simulink model "MotorSpeedAnalysisLAST"  (R2016a)
settings: Solver=ode4  SolverMode=SingleTasking  StartTime=0.0  StopTime=10  FixedStep=Ts  RelTol=1e-3
undefined symbols (not defined in the file): Ts
libraries: arduino_io_lib x4, powerlib_meascontrol x1
settings Model: ExtModeTrigDuration=2  Creator=gcampa  LastModifiedBy=User
settings DataIOCC: LimitDataPoints=on  SaveFormat=Array  SignalLoggingSaveFormat=ModelDataLogs
settings OptimizationCC: OptimizeModelRefInitCode=on  LifeSpan=1  MaxStackSize=64
settings DebuggingCC: UnderspecifiedInitializationDetection=Classic  MergeDetectMultiDrivingBlocksExec=none  MultiTaskDSMMsg=warning  MultiTaskCondExecSysMsg=none
settings HardwareCC: ProdBitPerInt=16  ProdBitPerPointer=16  ProdLargestAtomicFloat=None  ProdWordSize=8  ProdHWDeviceType=Atmel->AVR
settings ModelReferenceCC: PropagateSignalLabelsOutOfModel=off
settings RTWCC: SystemTargetFile=ert.tlc  HardwareBoard=Arduino Uno  TemplateMakefile=ert_default_tmf  GenerateReport=on  RTWVerbose=off  Toolchain=Arduino AVR v1.6.1  BuildConfiguration=Faster Runs  IncludeHyperlinkInReport=on  LaunchReport=on  GenerateTraceInfo=on  GenerateTraceReport=on  GenerateTraceReportSl=on  GenerateTraceReportSf=on  GenerateTraceReportEml=on
settings CodeAppCC: ForceParamTrailComments=on  IgnoreCustomStorageClasses=off  OperatorAnnotations=on  SimulinkDataObjDesc=on  SFDataObjDesc=on  MATLABFcnDesc=on  InsertBlockDesc=on  MATLABSourceComments=on
settings ERTTargetCC: SupportContinuousTime=on  SupportVariableSizeSignals=on
settings ConfigComp: CovModelRefEnable=Off

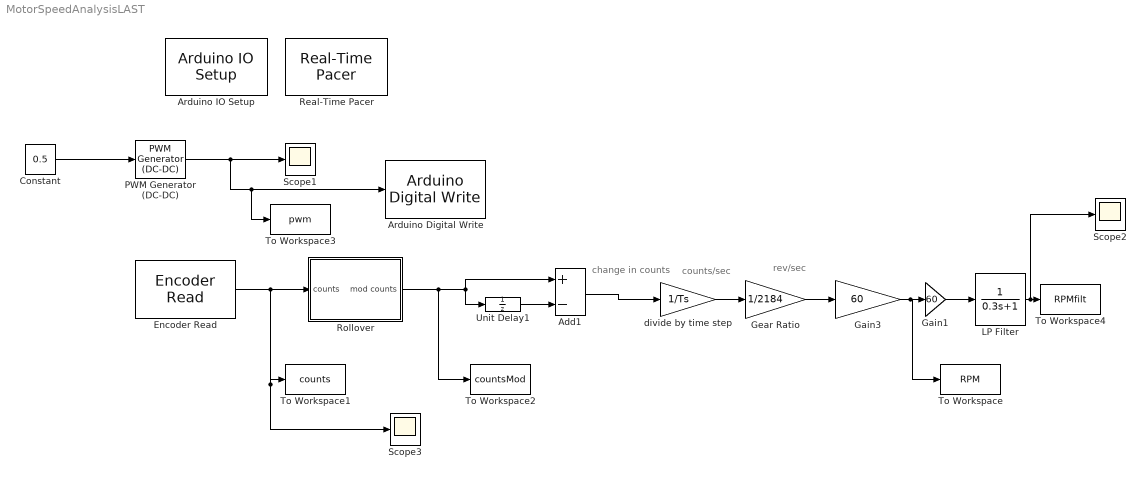
== system MotorSpeedAnalysisLAST ==
  note: change
      | in counts
  note: rev/sec
  note: counts/sec
  Add1 : Sum  Inputs=+-
  Arduino Digital Write : arduino_io_lib/Arduino Digital Write  arduinoVar=Temporary arduino variable: Arduino1  arduinoPin=5  T=-1
  Arduino IO Setup : arduino_io_lib/Arduino IO Setup  Priority=3  arduinoVar=Temporary arduino variable: Arduino1  workspaceVarName=b  comPort=COM4
  Constant : Constant  Value=0.5
  Encoder Read : arduino_io_lib/Encoder Read  arduinoVar=Temporary arduino variable: Arduino1  encNum=2  pinA=3  pinB=2  DbDl=0  T=Ts
  Gain1 : Gain  Gain=60
  Gain3 : Gain  Gain=60
  Gear Ratio : Gain  Gain=1/2184
  LP Filter : TransferFcn  Denominator=[0.3 1]
  PWM Generator (DC-DC) : powerlib_meascontrol/Pulse & Signal Generators/PWM Generator (DC-DC)  Fsw=10  Ts=Ts
  Real-Time Pacer : arduino_io_lib/Real-Time Pacer  simTimePerRealTime=1
  Rollover : Subsystem
  Scope1 : Scope
  Scope2 : Scope
  Scope3 : Scope
  To Workspace : ToWorkspace  VariableName=RPM  SaveFormat=Timeseries  SampleTime=-1
  To Workspace1 : ToWorkspace  VariableName=counts  SaveFormat=Timeseries  SampleTime=-1
  To Workspace2 : ToWorkspace  VariableName=countsMod  SaveFormat=Timeseries  SampleTime=-1
  To Workspace3 : ToWorkspace  VariableName=pwm  SaveFormat=Timeseries  SampleTime=-1
  To Workspace4 : ToWorkspace  VariableName=RPMfilt  SaveFormat=Timeseries  SampleTime=-1
  Unit Delay1 : UnitDelay  SampleTime=-1
  divide by time step : Gain  Gain=1/Ts
  wires:
  Unit Delay1/1 -> Add1/2
  Gear Ratio/1 -> Gain3/1
  divide by time step/1 -> Gear Ratio/1
  Add1/1 -> divide by time step/1
  Rollover/1(" mod counts") -> To Workspace2/1, Add1/1, Unit Delay1/1
  Encoder Read/1 -> Scope3/1, To Workspace1/1, Rollover/1(counts)
  Gain3/1 -> To Workspace/1, Gain1/1
  Constant/1 -> PWM Generator (DC-DC)/1
  PWM Generator (DC-DC)/1 -> To Workspace3/1, Arduino Digital Write/1, Scope1/1
  Gain1/1 -> LP Filter/1
  LP Filter/1 -> Scope2/1, To Workspace4/1

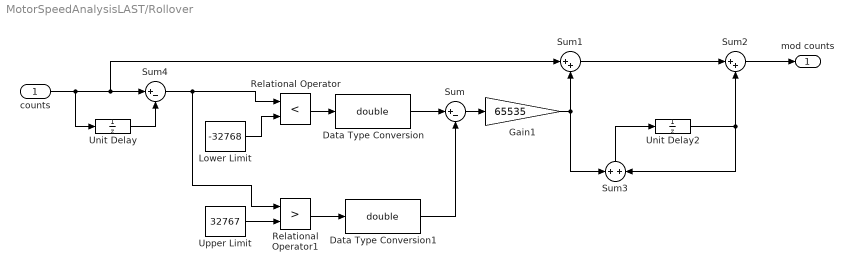
== system MotorSpeedAnalysisLAST/Rollover ==
  counts : Inport
  " Lower Limit" : Constant  Value=-32768
  " Upper Limit" : Constant  Value=32767
  Data Type Conversion : DataTypeConversion  OutDataTypeStr=double  RndMeth=Zero
  Data Type Conversion1 : DataTypeConversion  OutDataTypeStr=double  RndMeth=Zero
  Gain1 : Gain  Gain=65535
  Relational Operator : RelationalOperator  Operator=<  OutDataTypeStr=boolean
  Relational Operator1 : RelationalOperator  Operator=>  OutDataTypeStr=boolean
  Sum : Sum  Inputs=|+-
  Sum1 : Sum  Inputs=|++
  Sum2 : Sum  Inputs=|++
  Sum3 : Sum
  Sum4 : Sum  Inputs=|+-
  Unit Delay : UnitDelay  SampleTime=-1
  Unit Delay2 : UnitDelay  SampleTime=-1
  " mod counts" : Outport
  wires:
  counts/1 -> Unit Delay/1, Sum1/1, Sum4/1
  Sum2/1 -> " mod counts"/1
  Unit Delay/1 -> Sum4/2
  Data Type Conversion/1 -> Sum/1
  Sum3/1 -> Unit Delay2/1
  Data Type Conversion1/1 -> Sum/2
  Sum/1 -> Gain1/1
  Gain1/1 -> Sum1/2, Sum3/1
  Relational Operator1/1 -> Data Type Conversion1/1
  Sum1/1 -> Sum2/1
  Relational Operator/1 -> Data Type Conversion/1
  " Upper Limit"/1 -> Relational Operator1/2
  Unit Delay2/1 -> Sum3/2, Sum2/2
  " Lower Limit"/1 -> Relational Operator/2
  Sum4/1 -> Relational Operator/1, Relational Operator1/1
